simulink model "Dynamic_Braking_with_Variable_Resistors"  (R2024b)
settings: Solver=VariableStepAuto  StartTime=0.0  StopTime=2.2  RelTol=1e-3
values from neighbouring files (symbols this model uses):
  R1 = 10    [Dynamic_Braking_with_Variable_Resistors.m]
  R2 = 20    [Dynamic_Braking_with_Variable_Resistors.m]
  R3 = 40    [Dynamic_Braking_with_Variable_Resistors.m]
  Va = 220    [Dynamic_Braking_with_Variable_Resistors.m]
undefined symbols (not defined in the file or in its folder): RPM, sigbuilder_block, T, Vf
libraries: spsIdealSwitchLib x5, spsSeriesRLCBranchLib x3, spsDCVoltageSourceLib x2, spsCurrentMeasurementLib x1, spsDCMachineLib x1, spsGroundLib x1, sps_lib x1
settings Model: Creator=aayus  LastModifiedBy=aayus

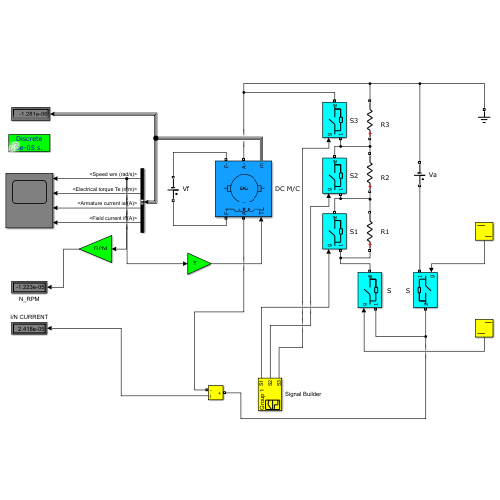
[thumbnail: Simulink's stored preview of the top-level diagram]
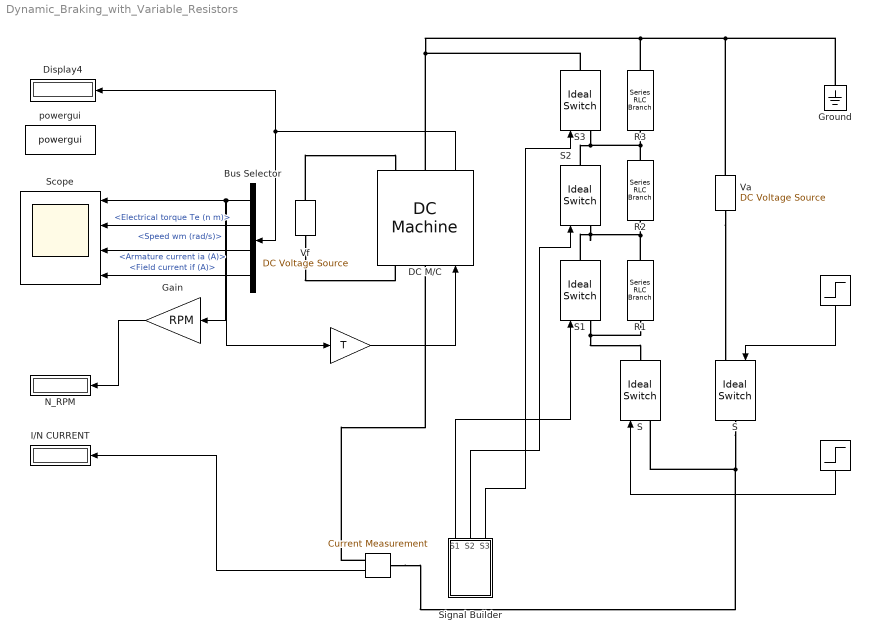
== system Dynamic_Braking_with_Variable_Resistors ==
  " R2" : spsSeriesRLCBranchLib/Series RLC Branch  LConnTagsString=__new0  RConnTagsString=__new0  BranchType=R  Resistance=R2  Inductance=1e-3  SetiL0=off  InitialCurrent=0  Capacitance=1e-6  Setx0=off  InitialVoltage=0  Measurements=None
  " R3" : spsSeriesRLCBranchLib/Series RLC Branch  LConnTagsString=__new0  RConnTagsString=__new0  BranchType=R  Resistance=R3  Inductance=1e-3  SetiL0=off  InitialCurrent=0  Capacitance=1e-6  Setx0=off  InitialVoltage=0  Measurements=None
  " " : Step  Before=1  After=0  SampleTime=0
  "  " : Step  SampleTime=0
  "   " : spsCurrentMeasurementLib/Current Measurement  PhasorSimulation=off  OutputType=Complex  PSBequivalent=0
  "     " : Gain  Gain=T
  " S" : spsIdealSwitchLib/Ideal Switch  Ron=0.001  Lon=0  IC=0  Rs=1e5  Cs=inf  Measurements=off
  Bus Selector : BusSelector  OutputSignals=Speed wm (rad/s),Electrical torque Te (n m),Armature current ia (A),Field current if (A)
  DC M/C : spsDCMachineLib/DC Machine  PresetModel=No  MechanicalLoad=Torque TL  FieldType=Wound  ShowDetailedParameters=on  MeasurementBus=off  RLa=[0.5 0.02]  RLf=[150 112.5]  Laf=1.234  MachineConstant=Torque constant (N.m/A)  Ke=1.8  Kt=1.8  J=0.1  Bm=0.008  Tf=0.006  w0=1  Ifinit=1  TsPowergui=0  TsBlock=-1
  Display4 : Display
  Gain : Gain  Gain=RPM
  Ground : spsGroundLib/Ground  LConnTagsString=a
  I/N CURRENT : Display
  N_RPM : Display
  R1 : spsSeriesRLCBranchLib/Series RLC Branch  LConnTagsString=__new0  RConnTagsString=__new0  BranchType=R  Resistance=R1  Inductance=1e-3  SetiL0=off  InitialCurrent=0  Capacitance=1e-6  Setx0=off  InitialVoltage=0  Measurements=None
  S{,1..3} (4 alike) : spsIdealSwitchLib/Ideal Switch  Ron=0.001  Lon=0  IC=0  Rs=1e5  Cs=inf  Measurements=off
  Scope : Scope  NumInputPorts=4
  Signal Builder : Subsystem  Tag=STV Subsys  LoadFcn=sigbuilder_block('load');  StartFcn=sigbuilder_block('start');  StopFcn=sigbuilder_block('stop');  ClipboardFcn=sigbuilder_block('clipboard');  mask(Sigbuilder block){tuvar=[0:10]}
      mask help: Sigbuilder GUI
      mask init:
      | if ~strcmp(get_param(bdroot(gcbh),'SimulationStatus'),'stopped') tuvar = sigbuilder_block('maskInit'); end
      settings: CopyFcn=sigbuilder_block('copy');  DeleteFcn=sigbuilder_block('delete');  ModelCloseFcn=sigbuilder_block('modelClose');  PreSaveFcn=sigbuilder_block('preSave');  PauseFcn=sigbuilder_block('pause')  ContinueFcn=sigbuilder_block('continue')  NameChangeFcn=sigbuilder_block('namechange');  OpenFcn=sigbuilder_block('open',[257.25 56.25 705.75 447.75 ]);  CloseFcn=sigbuilder_block('close');
      mask Display: plot(0, 0, 100, 100,[2, 2, 32, 32, 2], [68, 8, 8, 68, 68],[32, 2], [38, 38], [32, 19, 2],[53, 60, 44], [32, 17, 17, 2],[16, 16, 31, 31]);txt = getActiveGroup(gcbh);text(2, 100, txt,'verticalAlignment', 'top');
  Va : spsDCVoltageSourceLib/DC Voltage Source  Amplitude=Va  Measurements=None
  Vf : spsDCVoltageSourceLib/DC Voltage Source  Amplitude=Vf  Measurements=None
  powergui : sps_lib/powergui  SimulationMode=Discrete  SampleTime=50e-6  frequency=60  Iterations=50  frequencyindice=0  Pbase=100e6  ErrMax=1e-4  UnitsV=kV  UnitsW=MW  buscounter=0  FunctionMessages=off  echomessages=off  EnableUseOfTLC=off  CurrentSourceSwitches=off  DisableSnubberDevices=off  DisableRonSwitches=off  DisableVfSwitches=off  DisplayEquations=off  AutomaticDiscreteSolvers=off  SolverType=Tustin/Backward Euler (TBE)  Interpol=off  ExternalGateDelay=off  methode=off  Ts=100  x0status=blocks  SPID=on  SwTol=0  HookPort=off  NonlinearTolerance=1e-4  nMaxIteration=100  ContinueOnMaxIteration=off  RestoreLinks=warning  ResistiveCurrentMeasurement=off  Frange=[0:2:500]  Ylog=off  Xlog=on  ShowGrid=off  save=off  variable=ZData  structure=0  ZoomFFT=on  StartTime=0.0  cycles=1  DisplayStyle=1  fundamental=60  FreqAxis=off  MaxFrequency=1000  frequencyindicesteady=1  RmsSteady=1  display=off
  wires:
  Signal Builder/1(S1) -> S1/1
  "   "/1 -> I/N CURRENT/1
  DC M/C/1 -> Bus Selector/1, Display4/1
  "     "/1 -> DC M/C/1
  Bus Selector/2 -> Scope/2  "<Electrical torque Te (n m)>"
  Signal Builder/3(S3) -> S3/1
  Bus Selector/1 -> Gain/1, Scope/1, "     "/1  "<Speed wm (rad/s)>"
  Signal Builder/2(S2) -> S2/1
  "  "/1 -> " S"/1
  Gain/1 -> N_RPM/1
  " "/1 -> S/1
  Bus Selector/3 -> Scope/3  "<Armature current ia (A)>"
  Bus Selector/4 -> Scope/4  "<Field current if (A)>"
  connections:
  " R3"/LConn1 -- S3/LConn1 -- S2/RConn1 -- " R2"/RConn1
  S/RConn1 -- "   "/LConn1 -- " S"/LConn1
  S1/RConn1 -- S2/LConn1 -- R1/RConn1 -- " R2"/LConn1
  DC M/C/RConn1 -- Va/LConn1 -- Ground/LConn1 -- " R3"/RConn1 -- S3/RConn1
  " S"/RConn1 -- S1/LConn1 -- R1/LConn1
  Vf/RConn1 -- DC M/C/LConn2
  Va/RConn1 -- S/LConn1
  "   "/RConn1 -- DC M/C/LConn1
  Vf/LConn1 -- DC M/C/RConn2

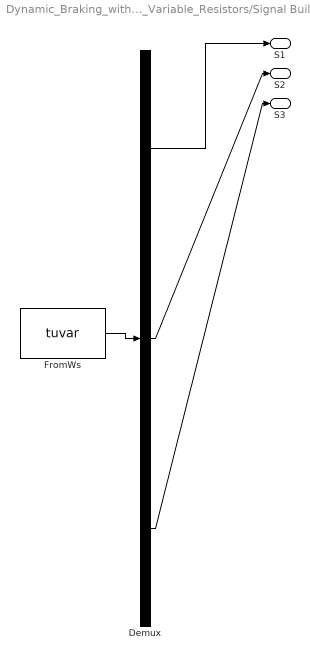
== system Dynamic_Braking_with_Variable_Resistors/Signal Builder ==
  Demux : Demux  Tag=STV Demux  Outputs=3
      settings: DisplayOption=none
  FromWs : FromWorkspace  Tag=STV FromWs  VariableName=tuvar
      SigBuilderData=|
      | common.afterFinalStr = 'Extrapolate'
      | common.sampleTime = 0
      | dataSet.timeRange = [0 10]
      | dataSet.name = 'Group 1'
      | sbobj.Name = 'Signal Builder'
      | sbobj.Groups.Name = 'Group 1'
      | sbobj.Groups.Signals(1).Name = 'S1'
      | sbobj.Groups.Signals(1).XData = [0 0.02 1.1 1.1 10]
      | sbobj.Groups.Signals(1).YData = [0 0 0 1 1]
      | sbobj.Groups.Signals(2).Name = 'S2'
      | sbobj.Groups.Signals(2).XData = [0 1.1 1.1 1.2 1.2 10]
      | sbobj.Groups.Signals(2).YData = [1 1 0 0 1 1]
      | sbobj.Groups.Signals(3).Name = 'S3'
      | sbobj.Groups.Signals(3).XData = [0 1.2 1.2 1.3 1.3 10]
      | sbobj.Groups.Signals(3).YData = [1 1 0 0 1 1]
  S1 : Outport  Tag=STV Outport
  S2 : Outport  Tag=STV Outport  Port=2
  S3 : Outport  Tag=STV Outport  Port=3
  wires:
  Demux/1 -> S1/1
  FromWs/1 -> Demux/1
  Demux/2 -> S2/1
  Demux/3 -> S3/1
